simulink model "PID_Interactive_3"  (R2017a)
settings: Solver=FixedStepDiscrete  StartTime=0.0  StopTime=10.0  FixedStep=.001  RelTol=1e-3
libraries: stellaris_lp_lib x11, simulink x6, xpcutilitieslib x2
settings Model: ExtModeTrigDuration=8  Creator=peselnikmg  LastModifiedBy=dhastin
settings DataIOCC: LimitDataPoints=on  SaveFormat=Array  SignalLoggingSaveFormat=ModelDataLogs  ReturnWorkspaceOutputs=on
settings OptimizationCC: UseDivisionForNetSlopeComputation=on  UseFloatMulNetSlope=on  DefaultUnderspecifiedDataType=single  UseSpecifiedMinMax=on  PassReuseOutputArgsAs=Individual arguments  ExpressionDepthLimit=2147483647  ZeroExternalMemoryAtStartup=off  NoFixptDivByZeroProtection=on  EfficientFloat2IntCast=on  LifeSpan=inf  MaxStackSize=64  OptimizeBlockOrder=speed
settings DebuggingCC: ReadBeforeWriteMsg=DisableAll  WriteAfterWriteMsg=DisableAll  WriteAfterReadMsg=DisableAll  MultiTaskDSMMsg=none  IntegerOverflowMsg=error  ParameterTunabilityLossMsg=error  AssertControl=DisableAll  StateNameClashWarn=warning  NonBusSignalsTreatedAsBus=error  SFInvalidInputDataAccessInChartInitDiag=error  SFTransitionOutsideNaturalParentDiag=error  SFUnreachableExecutionPathDiag=error  SFUndirectedBroadcastEventsDiag=error  SFExecutionAtInitializationDiag=none  IntegerSaturationMsg=error
settings HardwareCC: ProdBitPerPointer=32  ProdBitPerSizeT=32  ProdBitPerPtrDiffT=32  ProdLargestAtomicInteger=Long  ProdLargestAtomicFloat=Double  ProdWordSize=32  ProdHWDeviceType=ARM Compatible->ARM Cortex
settings ModelReferenceCC: UpdateModelReferenceTargets=IfOutOfDate  PropagateSignalLabelsOutOfModel=off
settings SFSimCC: SFSimEcho=off  MATLABDynamicMemAlloc=off
settings RTWCC: SystemTargetFile=ert.tlc  HardwareBoard=Tiva TM4C123G Launchpad  TLCOptions=-aInlineSetEventsForThisBaseRateFcn=TLC_FALSE -aSuppressMultiTaskScheduler=TLC_FALSE -aRateBasedStepFcn=1  TemplateMakefile=ert_default_tmf  Description=Embedded Coder  GenerateReport=on  RTWVerbose=off  Toolchain=Texas Instruments Code Composer Studio (Tiva)  IncludeHyperlinkInReport=on  LaunchReport=on  GenerateTraceInfo=on  GenerateTraceReport=on  GenerateTraceReportSl=on  GenerateTraceReportSf=on  GenerateTraceReportEml=on
settings CodeAppCC: ForceParamTrailComments=on  IgnoreCustomStorageClasses=off  OperatorAnnotations=on  SimulinkDataObjDesc=on  SFDataObjDesc=on  MATLABFcnDesc=on  CustomSymbolStrType=$N$R$M  InsertBlockDesc=on  MATLABSourceComments=on  EnableCustomComments=on  ReqsInCode=on
settings ERTTargetCC: UtilityFuncGeneration=Shared location  CombineSignalStateStructs=on  SuppressErrorStatus=on  SupportNonFinite=off  ParenthesesLevel=Maximum  CastingMode=Standards  EnableSignedLeftShifts=off  EnableSignedRightShifts=off
settings ConfigComp: CovMetricSettings=dw  CovHtmlReporting=on  CovSaveCumulativeToWorkspaceVar=on  CovSaveSingleToWorkspaceVar=on  CovExternalEMLEnable=off

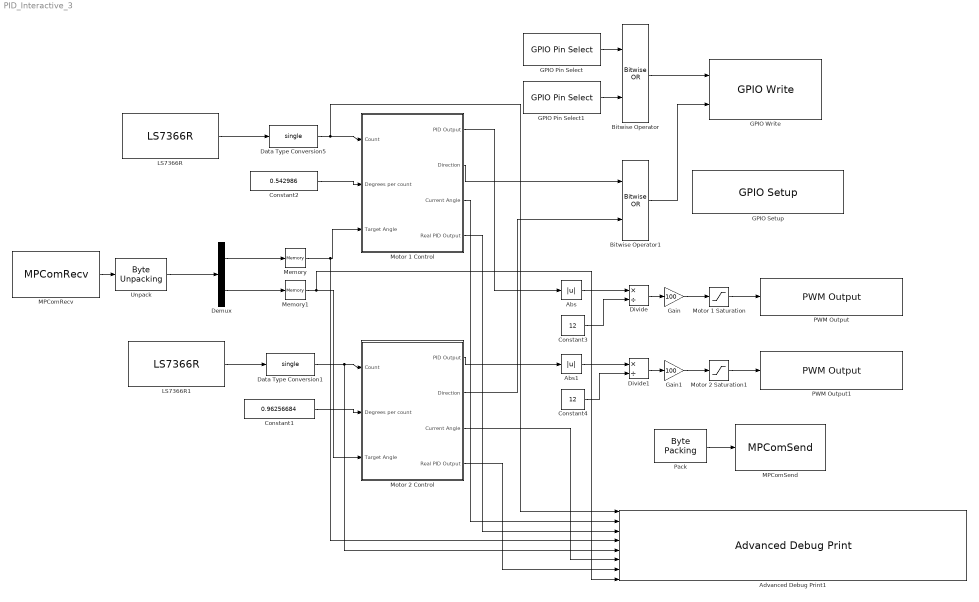
== system PID_Interactive_3 ==
  Abs : Abs
  Abs1 : Abs
  Advanced Debug Print1 : stellaris_lp_lib/Debug/Advanced Debug Print  types={'single','single','single','single','single','single','single','single'}  fmt='\nM1C %hf A %hf PID %hf RxA %hf\n\rM2C %hf A %hf PID %hf RxA %hf\r\n\n'  sample_time=0.1
      settings: SourceProductName=Run on Stellaris LaunchPad
  Bitwise Operator : simulink/Logic and Bit Operations/Bitwise Operator  logicop=OR  UseBitMask=off  NumInputPorts=2  BitMask=bin2dec('11011001')  BitMaskRealWorld=Stored Integer
  Bitwise Operator1 : simulink/Logic and Bit Operations/Bitwise Operator  logicop=OR  UseBitMask=off  NumInputPorts=2  BitMask=bin2dec('11011001')  BitMaskRealWorld=Stored Integer
  Constant1 : Constant  Value=0.96256684  OutDataTypeStr=single  LockScale=on
  Constant2 : Constant  Value=0.542986  OutDataTypeStr=single  LockScale=on
  Constant3 : Constant  Value=12  OutDataTypeStr=single  LockScale=on
  Constant4 : Constant  Value=12  OutDataTypeStr=single  LockScale=on
  Data Type Conversion1 : DataTypeConversion  OutDataTypeStr=single
  Data Type Conversion5 : DataTypeConversion  OutDataTypeStr=single
  Demux : Demux  Outputs=2
  Divide : Product  Inputs=*/
  Divide1 : Product  Inputs=*/
  GPIO Pin Select : stellaris_lp_lib/GPIO/GPIO Pin Select  GPIO_PIN_X=GPIO_PIN_2
      settings: SourceProductName=Run on Stellaris LaunchPad
  GPIO Pin Select1 : stellaris_lp_lib/GPIO/GPIO Pin Select  GPIO_PIN_X=GPIO_PIN_3
      settings: SourceProductName=Run on Stellaris LaunchPad
  GPIO Setup : stellaris_lp_lib/GPIO/GPIO Setup  GPIO_PORTX_BASE=GPIO_PORTF_BASE  PinsOutput_0=Unused  PinsOutput_1=Unused  PinsOutput_2=Output  PinsOutput_3=Output  PinsOutput_4=Unused  PinsOutput_5=Unused  PinsOutput_6=Unused  PinsOutput_7=Unused
      settings: SourceProductName=Run on Stellaris LaunchPad
  GPIO Write : stellaris_lp_lib/GPIO/GPIO Write  GPIO_PORTX_BASE=GPIO_PORTF_BASE  SampleTime=-1
      settings: SourceProductName=Run on Stellaris LaunchPad
  Gain : Gain  Gain=100
  Gain1 : Gain  Gain=100
  LS7366R : stellaris_lp_lib/SPIDev/LS7366R  ssel="CH 1  (SSEL: PA3)"  ext_clk=on  sample_time=-1
      settings: SourceProductName=Run on Stellaris LaunchPad
  LS7366R1 : stellaris_lp_lib/SPIDev/LS7366R  ssel="CH 2  (SSEL: PD0)"  ext_clk=on  sample_time=-1
      settings: SourceProductName=Run on Stellaris LaunchPad
  MPComRecv : stellaris_lp_lib/Communication/MPComRecv  vport=2  pack_size=8  sample_time=-1
      settings: SourceProductName=Run on Stellaris LaunchPad
  MPComSend : stellaris_lp_lib/Communication/MPComSend  vport=3  pack_size=8  sample_time=-1
      settings: SourceProductName=Run on Stellaris LaunchPad
  Memory : Memory
  Memory1 : Memory
  Motor 1 Saturation : Saturate  UpperLimit=95  LowerLimit=0
  Motor 1 Control : Subsystem
  Motor 2 Saturation1 : Saturate  UpperLimit=95  LowerLimit=0
  Motor 2 Control : Subsystem
  PWM Output : stellaris_lp_lib/PWM/PWM Output  ch="1    PC4"  invert=off  freq=22000  sample_time=-1
      settings: SourceProductName=Run on Stellaris LaunchPad
  PWM Output1 : stellaris_lp_lib/PWM/PWM Output  ch="2    PC5"  invert=off  freq=22000  sample_time=-1
      settings: SourceProductName=Run on Stellaris LaunchPad
  Pack : xpcutilitieslib/Byte Packing   MaskPackedDataType=uint8  MaskUnpackedDataTypes={'single','single'}  MaskAlignment=1
  Unpack : xpcutilitieslib/Byte Unpacking   MaskUnpackedDataTypes={['single']}  MaskUnpackedDataSizes={[1,2]}  MaskAlignment=1
      settings: SourceProductName=Simulink Real-Time  SourceProductBaseCode=XP
  wires:
  MPComRecv/1 -> Unpack/1
  Demux/2 -> Memory1/1
  Pack/1 -> MPComSend/1
  Unpack/1 -> Demux/1
  Memory/1 -> Advanced Debug Print1/4, Motor 1 Control/3(Target Angle)
  Demux/1 -> Memory/1
  LS7366R/1 -> Data Type Conversion5/1
  Data Type Conversion5/1 -> Advanced Debug Print1/1, Motor 1 Control/1(Count)
  GPIO Pin Select/1 -> Bitwise Operator/1
  GPIO Pin Select1/1 -> Bitwise Operator/2
  Bitwise Operator/1 -> GPIO Write/1
  Bitwise Operator1/1 -> GPIO Write/2
  Constant2/1 -> Motor 1 Control/2(Degrees per count)
  Motor 1 Control/2(Direction) -> Bitwise Operator1/1
  Memory1/1 -> Advanced Debug Print1/8, Motor 2 Control/3(Target Angle)
  LS7366R1/1 -> Data Type Conversion1/1
  Data Type Conversion1/1 -> Advanced Debug Print1/5, Motor 2 Control/1(Count)
  Constant1/1 -> Motor 2 Control/2(Degrees per count)
  Motor 1 Control/1(PID Output) -> Abs/1
  Motor 2 Saturation1/1 -> PWM Output1/1
  Motor 2 Control/1(PID Output) -> Abs1/1
  Motor 2 Control/2(Direction) -> Bitwise Operator1/2
  Motor 2 Control/3(Current Angle) -> Advanced Debug Print1/6
  Motor 1 Control/3(Current Angle) -> Advanced Debug Print1/2
  Divide/1 -> Gain/1
  Abs/1 -> Divide/1
  Constant3/1 -> Divide/2
  Motor 1 Saturation/1 -> PWM Output/1
  Divide1/1 -> Gain1/1
  Abs1/1 -> Divide1/1
  Constant4/1 -> Divide1/2
  Gain/1 -> Motor 1 Saturation/1
  Gain1/1 -> Motor 2 Saturation1/1
  Motor 1 Control/4("Real PID Output ") -> Advanced Debug Print1/3
  Motor 2 Control/4(Real PID Output) -> Advanced Debug Print1/7

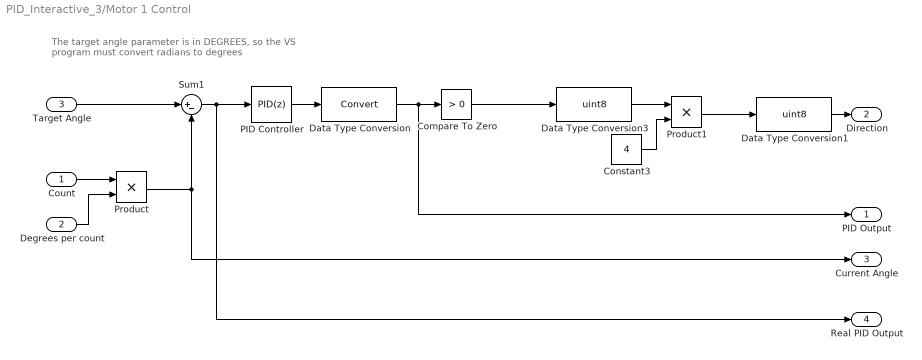
== system PID_Interactive_3/Motor 1 Control ==
  note: The target angle parameter is in DEGREES, so the VS program must convert radians to degrees
  Count : Inport
  Degrees per count : Inport  Description=Degrees per tick  Port=2
  Target Angle : Inport  Port=3
  Compare To Zero : simulink/Logic and Bit Operations/Compare To Zero  relop=>  OutDataTypeStr=boolean
  Constant3 : Constant  Value=4  OutDataTypeStr=uint8
  Data Type Conversion : DataTypeConversion
  Data Type Conversion1 : DataTypeConversion  OutDataTypeStr=uint8
  Data Type Conversion3 : DataTypeConversion  OutDataTypeStr=uint8
  PID Controller : simulink/Continuous/PID Controller  Controller=PID  TimeDomain=Discrete-time  SampleTime=-1  IntegratorMethod=Forward Euler  FilterMethod=Forward Euler  Form=Parallel  UseFilter=on  ControllerParametersSource=internal  P=10  I=0  D=0  N=20  InitialConditionSource=internal  InitialConditionForIntegrator=0  InitialConditionForFilter=0  ExternalReset=none  LimitOutput=on  UpperSaturationLimit=12  LowerSaturationLimit=-12  LinearizeAsGain=on  AntiWindupMode=clamping  Kb=1  TrackingMode=off  Kt=1  PParamMin=[]  PParamMax=[]  IParamMin=[]  IParamMax=[]  DParamMin=[]  DParamMax=[]  NParamMin=[]  NParamMax=[]  KbParamMin=[]  KbParamMax=[]  KtParamMin=[]  KtParamMax=[]  POutMin=[]  POutMax=[]  IOutMin=[]  IOutMax=[]  DOutMin=[]  DOutMax=[]  NOutMin=[]  NOutMax=[]  KbOutMin=[]  KbOutMax=[]  KtOutMin=[]  KtOutMax=[]  IntegratorOutMin=[]  IntegratorOutMax=[]  FilterOutMin=[]  FilterOutMax=[]  SumOutMin=[]  SumOutMax=[]  SumI1OutMin=[]  SumI1OutMax=[]  SumI2OutMin=[]  SumI2OutMax=[]  SumI3OutMin=[]  SumI3OutMax=[]  SumDOutMin=[]  SumDOutMax=[]  SaturationOutMin=[]  SaturationOutMax=[]  IntegratorContinuousStateAttributes=''  IntegratorStateMustResolveToSignalObject=off  IntegratorRTWStateStorageClass=Auto  FilterContinuousStateAttributes=''  FilterStateMustResolveToSignalObject=off  FilterRTWStateStorageClass=Auto  DifferentiatorICPrevScaledInput=0  DifferentiatorOutMin=[]  DifferentiatorOutMax=[]  InitialConditionSetting=State (most efficient)
  Product : Product  OutDataTypeStr=single
  Product1 : Product  OutDataTypeStr=single
  Sum1 : Sum  Inputs=|+-
  PID Output : Outport
  Direction : Outport  Port=2
  Current Angle : Outport  Port=3
  "Real PID Output " : Outport  Port=4
  wires:
  Data Type Conversion/1 -> PID Output/1, Compare To Zero/1
  Constant3/1 -> Product1/2
  Sum1/1 -> "Real PID Output "/1, PID Controller/1
  Degrees per count/1 -> Product/2
  Data Type Conversion3/1 -> Product1/1
  Compare To Zero/1 -> Data Type Conversion3/1
  Product/1 -> Current Angle/1, Sum1/2
  PID Controller/1 -> Data Type Conversion/1
  Data Type Conversion1/1 -> Direction/1
  Count/1 -> Product/1
  Target Angle/1 -> Sum1/1
  Product1/1 -> Data Type Conversion1/1

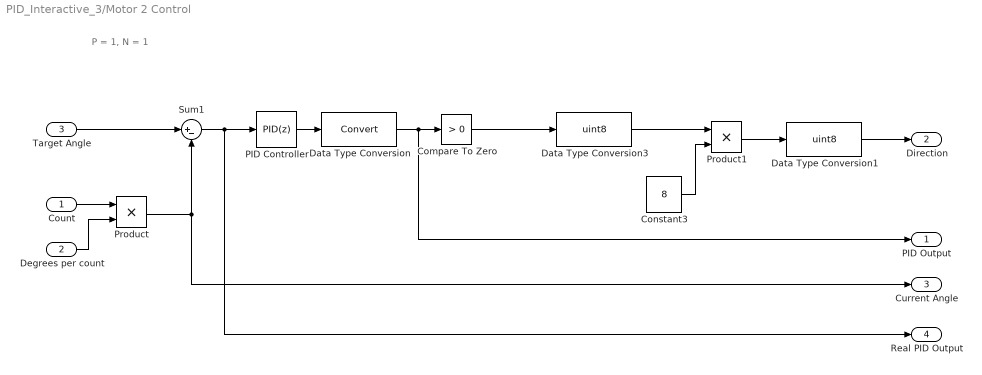
== system PID_Interactive_3/Motor 2 Control ==
  note: P = 1, N = 1
  Count : Inport
  Degrees per count : Inport  Description=Degrees per tick  Port=2
  Target Angle : Inport  Port=3
  Compare To Zero : simulink/Logic and Bit Operations/Compare To Zero  relop=>  OutDataTypeStr=boolean
  Constant3 : Constant  Value=8  OutDataTypeStr=uint8
  Data Type Conversion : DataTypeConversion
  Data Type Conversion1 : DataTypeConversion  OutDataTypeStr=uint8
  Data Type Conversion3 : DataTypeConversion  OutDataTypeStr=uint8
  PID Controller : simulink/Continuous/PID Controller  Controller=PID  TimeDomain=Discrete-time  SampleTime=-1  IntegratorMethod=Forward Euler  FilterMethod=Forward Euler  Form=Parallel  UseFilter=on  ControllerParametersSource=internal  P=4  I=0  D=0  N=20  InitialConditionSource=internal  InitialConditionForIntegrator=0  InitialConditionForFilter=0  ExternalReset=none  LimitOutput=on  UpperSaturationLimit=12  LowerSaturationLimit=-12  LinearizeAsGain=on  AntiWindupMode=clamping  Kb=1  TrackingMode=off  Kt=1  PParamMin=[]  PParamMax=[]  IParamMin=[]  IParamMax=[]  DParamMin=[]  DParamMax=[]  NParamMin=[]  NParamMax=[]  KbParamMin=[]  KbParamMax=[]  KtParamMin=[]  KtParamMax=[]  POutMin=[]  POutMax=[]  IOutMin=[]  IOutMax=[]  DOutMin=[]  DOutMax=[]  NOutMin=[]  NOutMax=[]  KbOutMin=[]  KbOutMax=[]  KtOutMin=[]  KtOutMax=[]  IntegratorOutMin=[]  IntegratorOutMax=[]  FilterOutMin=[]  FilterOutMax=[]  SumOutMin=[]  SumOutMax=[]  SumI1OutMin=[]  SumI1OutMax=[]  SumI2OutMin=[]  SumI2OutMax=[]  SumI3OutMin=[]  SumI3OutMax=[]  SumDOutMin=[]  SumDOutMax=[]  SaturationOutMin=[]  SaturationOutMax=[]  IntegratorContinuousStateAttributes=''  IntegratorStateMustResolveToSignalObject=off  IntegratorRTWStateStorageClass=Auto  FilterContinuousStateAttributes=''  FilterStateMustResolveToSignalObject=off  FilterRTWStateStorageClass=Auto  DifferentiatorICPrevScaledInput=0  DifferentiatorOutMin=[]  DifferentiatorOutMax=[]  InitialConditionSetting=State (most efficient)
  Product : Product  OutDataTypeStr=single
  Product1 : Product  OutDataTypeStr=single
  Sum1 : Sum  Inputs=|+-
  PID Output : Outport
  Direction : Outport  Port=2
  Current Angle : Outport  Port=3
  Real PID Output : Outport  Port=4
  wires:
  Data Type Conversion/1 -> PID Output/1, Compare To Zero/1
  Constant3/1 -> Product1/2
  Sum1/1 -> Real PID Output/1, PID Controller/1
  Degrees per count/1 -> Product/2
  Data Type Conversion3/1 -> Product1/1
  Product/1 -> Current Angle/1, Sum1/2
  PID Controller/1 -> Data Type Conversion/1
  Data Type Conversion1/1 -> Direction/1
  Count/1 -> Product/1
  Compare To Zero/1 -> Data Type Conversion3/1
  Target Angle/1 -> Sum1/1
  Product1/1 -> Data Type Conversion1/1
